simulink model "Project2Simulink"  (R2020a)
settings: Solver=VariableStepAuto  StartTime=0.0  StopTime=10.0  RelTol=1e-3
libraries: simulink x1
settings Model: Creator=cresp  LastModifiedBy=cresp

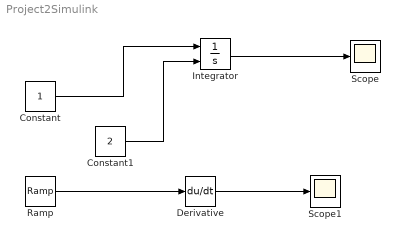
== system Project2Simulink ==
  Constant : Constant
  Constant1 : Constant  Value=2
  Derivative : Derivative
  Integrator : Integrator  InitialConditionSource=external  InitialCondition=2
  Ramp : simulink/Sources/Ramp  slope=1  start=0  InitialOutput=0
  Scope : Scope
  Scope1 : Scope
  wires:
  Constant/1 -> Integrator/1
  Integrator/1 -> Scope/1
  Derivative/1 -> Scope1/1
  Ramp/1 -> Derivative/1
  Constant1/1 -> Integrator/2
